simulink model "ShubhamGupta_180749_Lab7_4"  (R2020b)
settings: Solver=ode2  StartTime=0.0  StopTime=50  FixedStep=0.1  RelTol=1e-3
values from neighbouring files (symbols this model uses):
  TD = x(5)    [ShubhamGupta_180749_Lab7_ISTAE.m]
  TP = x(4)    [ShubhamGupta_180749_Lab7_ISTAE.m]
undefined symbols (not defined in the file or in its folder): ThetaD, ThetaP
settings Model: Creator=Nitin Kaistha  LastModifiedBy=subhamgupta
settings DataIOCC: ReturnWorkspaceOutputs=off

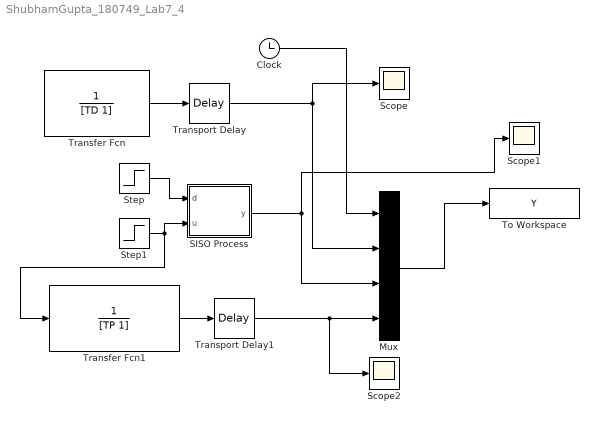
== system ShubhamGupta_180749_Lab7_4 ==
  Clock : Clock
  Mux : Mux
  SISO Process : Subsystem  mask{Kp=1, Tp=1, Kd=1, Td=3}
      mask prompts: Kp "Gp Gain"; Tp "Gp Time Constant"; Kd "Gd Gain"; Td "Gd Time Constant"
  Scope : Scope
  Scope1 : Scope
  Scope2 : Scope
  Step : Step  Time=0  After=0  SampleTime=0
  Step1 : Step  SampleTime=0
  To Workspace : ToWorkspace  VariableName=Y  SampleTime=-1
  Transfer Fcn : TransferFcn  Denominator=[TD 1]
  Transfer Fcn1 : TransferFcn  Denominator=[TP 1]
  Transport Delay : TransportDelay  DelayTime=ThetaD
  Transport Delay1 : TransportDelay  DelayTime=ThetaP
  wires:
  Step/1 -> SISO Process/1(d)
  Step1/1 -> Transfer Fcn1/1, SISO Process/2(u)
  Clock/1 -> Mux/1
  Mux/1 -> To Workspace/1
  Transfer Fcn/1 -> Transport Delay/1
  Transport Delay/1 -> Mux/2, Scope/1
  Transfer Fcn1/1 -> Transport Delay1/1
  Transport Delay1/1 -> Scope2/1, Mux/4
  SISO Process/1(y) -> Scope1/1, Mux/3

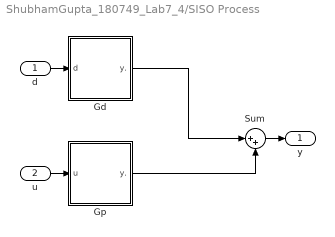
== system ShubhamGupta_180749_Lab7_4/SISO Process ==
  d : Inport
  u : Inport  Port=2
  Gd : Subsystem
  Gp : Subsystem
  Sum : Sum  Inputs=|++
  y : Outport
  wires:
  u/1 -> Gp/1(u)
  Gp/1(y.) -> Sum/2
  Sum/1 -> y/1
  Gd/1(y.) -> Sum/1
  d/1 -> Gd/1(d)

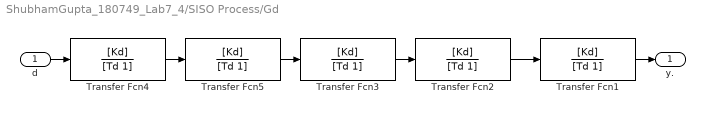
== system ShubhamGupta_180749_Lab7_4/SISO Process/Gd ==
  d : Inport
  Transfer Fcn{1..5} (5 alike) : TransferFcn  Numerator=[Kd]  Denominator=[Td 1]
  y. : Outport
  wires:
  Transfer Fcn4/1 -> Transfer Fcn5/1
  Transfer Fcn5/1 -> Transfer Fcn3/1
  d/1 -> Transfer Fcn4/1
  Transfer Fcn2/1 -> Transfer Fcn1/1
  Transfer Fcn3/1 -> Transfer Fcn2/1
  Transfer Fcn1/1 -> y./1

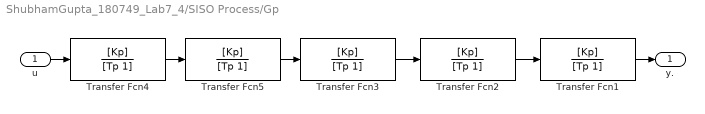
== system ShubhamGupta_180749_Lab7_4/SISO Process/Gp ==
  u : Inport
  Transfer Fcn{1..5} (5 alike) : TransferFcn  Numerator=[Kp]  Denominator=[Tp 1]
  y. : Outport
  wires:
  Transfer Fcn4/1 -> Transfer Fcn5/1
  Transfer Fcn5/1 -> Transfer Fcn3/1
  u/1 -> Transfer Fcn4/1
  Transfer Fcn2/1 -> Transfer Fcn1/1
  Transfer Fcn3/1 -> Transfer Fcn2/1
  Transfer Fcn1/1 -> y./1
